simulink model "STRbase"  (R2022a)
settings: Solver=VariableStepAuto  StartTime=0.0  StopTime=300  RelTol=1e-3
settings Model: Creator=user  LastModifiedBy=user

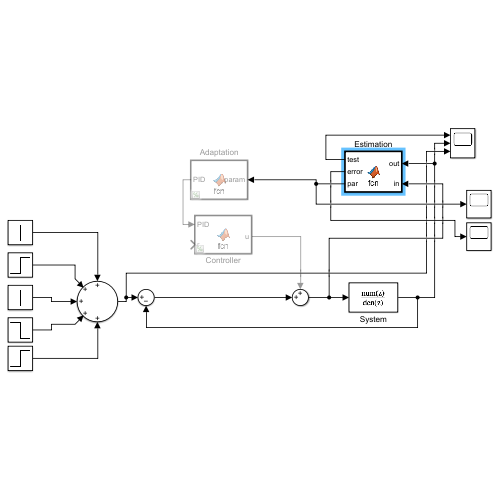
[thumbnail: Simulink's stored preview of the top-level diagram]
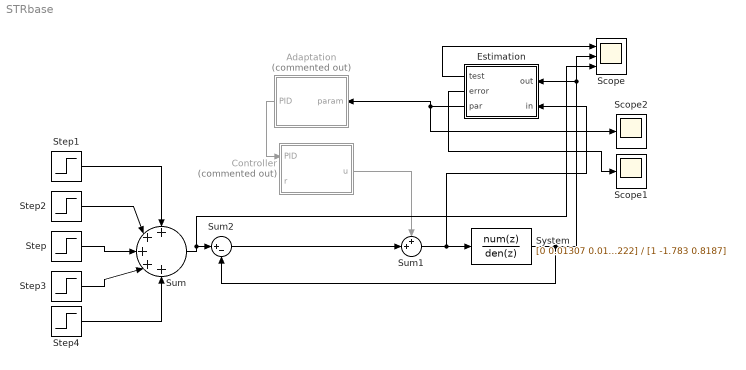
== system STRbase ==
  Adaptation : MATLAB Function  Commented=on  TreatAsAtomicUnit=on
  Controller : MATLAB Function  Commented=on  TreatAsAtomicUnit=on
  Estimation : MATLAB Function  TreatAsAtomicUnit=on
  Scope : Scope  NumInputPorts=3
  Scope1 : Scope
  Scope2 : Scope
  Step : Step  Time=50  After=2  SampleTime=0
  Step1 : Step  Time=80  After=-2  SampleTime=0
  Step2 : Step  Time=100  SampleTime=0
  Step3 : Step  Time=180  After=-1  SampleTime=0
  Step4 : Step  Time=240  After=2  SampleTime=0
  Sum : Sum  Inputs=+|+|+|+|+
  Sum1 : Sum  Inputs=++|
  Sum2 : Sum  Inputs=|+-
  System : DiscreteTransferFcn  Numerator=[0 0.01307 0.01222]  Denominator=[1 -1.783 0.8187]  InitialStates=10  SampleTime=0.5
  wires:
  System/1 -> Scope/2, Estimation/1(out), Sum2/2
  Estimation/1(test) -> Scope/1
  Sum1/1 -> Estimation/2(in), System/1
  Estimation/3(par) -> Adaptation/1(param), Scope2/1
  Step1/1 -> Sum/1
  Step/1 -> Sum/3
  Step2/1 -> Sum/2
  Adaptation/1(PID) -> Controller/1(PID)
  Controller/1(u) -> Sum1/1
  Sum/1 -> Scope/3, Sum2/1
  Sum2/1 -> Sum1/2
  Estimation/2(error) -> Scope1/1
  Step3/1 -> Sum/4
  Step4/1 -> Sum/5

== matlab function STRbase/Controller ==
  data: PID input; r input; u output
function u = fcn(PID, r)

u = PID();

== matlab function STRbase/Estimation ==
  data: out input; in input; test output; error output; par output
function [test,error,par] = fcn(out,in)
%untuk sekarang dibatasin cmn khusus identifikasi dengan orde 2
m=2;
n=2;
lbd=0.97;
persistent ind outd P W 

if isempty(P)
    P=eye(m+n);
end

if isempty(W)
    W=zeros(m+n,1);    
end

if isempty(ind);
    ind=zeros(m,1);
end

if isempty(outd)
    outd=zeros(n,1);
end

%RLS nya
%matrix parameter w mengikuti bentuk x
%x = [y(k-1) y(k-2) u(k-1) u(k-2)]'

%param w kalau di transfer function penjelasan ada di function block
%Adaptation
    x = [outd;ind];
    phi = P*x;
    g = phi/(lbd+x'*phi);
    o = W;
    y= o'*x;
    e = out-y;
    W= W+g*e;
    P = (P-g*x'*P)/lbd;

outd=[out;outd(1:1:end-1,:)];
ind=[in;ind(1:1:end-1,:)];

par=W;

%test output variabel apa aja, default nya output RLS yaitu y
test=y;
error=e;
end

== matlab function STRbase/Adaptation ==
  data: param input; PID output
function PID = fcn(param)
%parameternya ini dibagi jadi dua part
%anggap sistem diskrit dengan 
%NUM = [0 b1 b2]
%DEN = [1 a1 a2]

%param(1) itu koef -y(k-1) atau klo di DEN itu -a1 
%param(2) itu koef -y(k-2) atau klo di DEN itu -a2

%param(3) itu koef u(k-1) atau klo di DEN itu b1 
%param(4) itu koef u(k-2) atau klo di DEN itu b2

y = u;
